simulink model "followAndAvoidBlocksDeploy"  (R2016b)
settings: Solver=FixedStepAuto  StartTime=0.0  StopTime=10.0  RelTol=1e-3  EnableMultiTasking=on
libraries: legoev3lib x5, simulink x1
settings Model: ExtModeTrigDuration=2  Creator=Nexel  LastModifiedBy=Nexel
settings SolverCC: PositivePriorityOrder=on
settings OptimizationCC: MaxStackSize=64
settings DebuggingCC: ParameterTunabilityLossMsg=error
settings HardwareCC: ProdBitPerPointer=32  ProdBitPerSizeT=32  ProdBitPerPtrDiffT=32  ProdLargestAtomicInteger=Long  ProdWordSize=32  ProdHWDeviceType=ARM Compatible->ARM 9
settings RTWCC: SystemTargetFile=ert.tlc  HardwareBoard=LEGO MINDSTORMS EV3  TLCOptions="-aInlineSetEventsForThisBaseRateFcn=TLC_FALSE -aSuppressMultiTaskScheduler=TLC_FALSE  -aRateBasedStepFcn=0"  TemplateMakefile=ert_default_tmf  Description=Embedded Coder  GenerateReport=on  Toolchain=Sourcery G++ Lite v2009q3  IncludeHyperlinkInReport=on  LaunchReport=on  GenerateTraceInfo=on  GenerateTraceReport=on  GenerateTraceReportSl=on  GenerateTraceReportSf=on  GenerateTraceReportEml=on
settings CodeAppCC: ForceParamTrailComments=on  IgnoreCustomStorageClasses=off  OperatorAnnotations=on  SimulinkDataObjDesc=on  SFDataObjDesc=on  MATLABFcnDesc=on  InsertBlockDesc=on  MATLABSourceComments=on
settings ERTTargetCC: SupportContinuousTime=on  SupportVariableSizeSignals=on

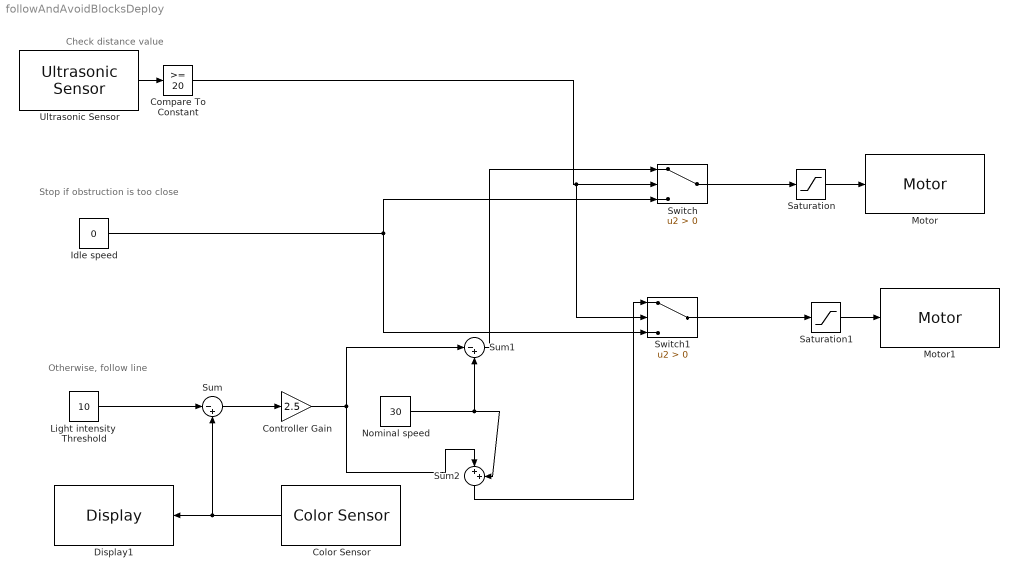
== system followAndAvoidBlocksDeploy ==
  note: Otherwise, follow line
  note: Stop if obstruction is too close
  note: Check distance value
  Color Sensor : legoev3lib/Color Sensor  portNumber=3  mode=Color  sampleTime=0.1
  Compare To Constant : simulink/Logic and Bit Operations/Compare To Constant  relop=>=  const=20  OutDataTypeStr=boolean
  "Controller Gain " : Gain  Gain=2.5
  Display1 : legoev3lib/Display  slcdLine=1  slcdFormat=Decimal
  "Idle speed " : Constant  Value=0
  "Light intensity  Threshold " : Constant  Value=10
  Motor : legoev3lib/Motor  sportNumber=B  sstopAction=Brake
  Motor1 : legoev3lib/Motor  sportNumber=C  sstopAction=Brake
  "Nominal speed " : Constant  Value=30
  Saturation : Saturate  UpperLimit=100  LowerLimit=-100
  Saturation1 : Saturate  UpperLimit=100  LowerLimit=-100
  Sum : Sum  Inputs=|-+
  Sum1 : Sum  Inputs=|-+
  Sum2 : Sum  Inputs=|++
  Switch : Switch  Criteria=u2 > Threshold
  Switch1 : Switch  Criteria=u2 > Threshold
  Ultrasonic Sensor : legoev3lib/Ultrasonic Sensor  PortNumber=4  sampleTime=0.1
  wires:
  "Light intensity  Threshold "/1 -> Sum/1
  Sum/1 -> "Controller Gain "/1
  Color Sensor/1 -> Display1/1, Sum/2
  "Controller Gain "/1 -> Sum2/1, Sum1/1
  "Nominal speed "/1 -> Sum2/2, Sum1/2
  Sum2/1 -> Switch1/1
  Sum1/1 -> Switch/1
  Ultrasonic Sensor/1 -> Compare To Constant/1
  "Idle speed "/1 -> Switch1/3, Switch/3
  Compare To Constant/1 -> Switch1/2, Switch/2
  Switch1/1 -> Saturation1/1
  Switch/1 -> Saturation/1
  Saturation/1 -> Motor/1
  Saturation1/1 -> Motor1/1
